simulink model "part2_3"  (R2018b)
settings: Solver=VariableStepAuto  StartTime=0.0  StopTime=1.0  RelTol=1e-3
libraries: simulink x2, dspsnks4 x1
settings Model: Creator=lisazaher  LastModifiedBy=lisazaher

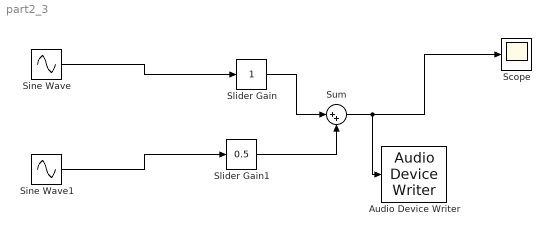
== system part2_3 ==
  Audio Device Writer : dspsnks4/Audio Device Writer  Driver=CoreAudio  Device=Default  InheritSampleRate=on  SampleRate=44100  BitDepth=16-bit integer  BufferSize=4096  NumBuffers=10  DefaultOutputChannelMapping=on  OutputChannelMapping=1:2  OutputNumUnderrunSamples=off  DriverIdx=5  DeviceWarnFlag=''
  Scope : Scope
  Sine Wave : Sin  SineType=Sample based  Samples=48  SampleTime=1/48000
  Sine Wave1 : Sin  SineType=Sample based  Samples=24  SampleTime=1/48000
  Slider Gain : simulink/Math Operations/Slider Gain  gain=1  low=0  high=2
  Slider Gain1 : simulink/Math Operations/Slider Gain  gain=0.5  low=0  high=1
  Sum : Sum  Inputs=|++
  wires:
  Sine Wave/1 -> Slider Gain/1
  Sine Wave1/1 -> Slider Gain1/1
  Slider Gain/1 -> Sum/1
  Slider Gain1/1 -> Sum/2
  Sum/1 -> Audio Device Writer/1, Scope/1
